simulink model "Simulering"  (R2021a)
settings: Solver=FixedStepDiscrete  StartTime=0.0  StopTime=100  FixedStep=0.0001  RelTol=1e-3
values from neighbouring files (symbols this model uses):
  D = 0.18    [grasklippare.m]
  L = 0.225    [grasklippare.m]
  r = 0.049    [grasklippare.m]
undefined symbols (not defined in the file or in its folder): DiscIntNeverNeededParam
libraries: simulink x4, pid_lib x3
settings Model: Creator=trane  LastModifiedBy=trane
settings SolverCC: AutoInsertRateTranBlk=on

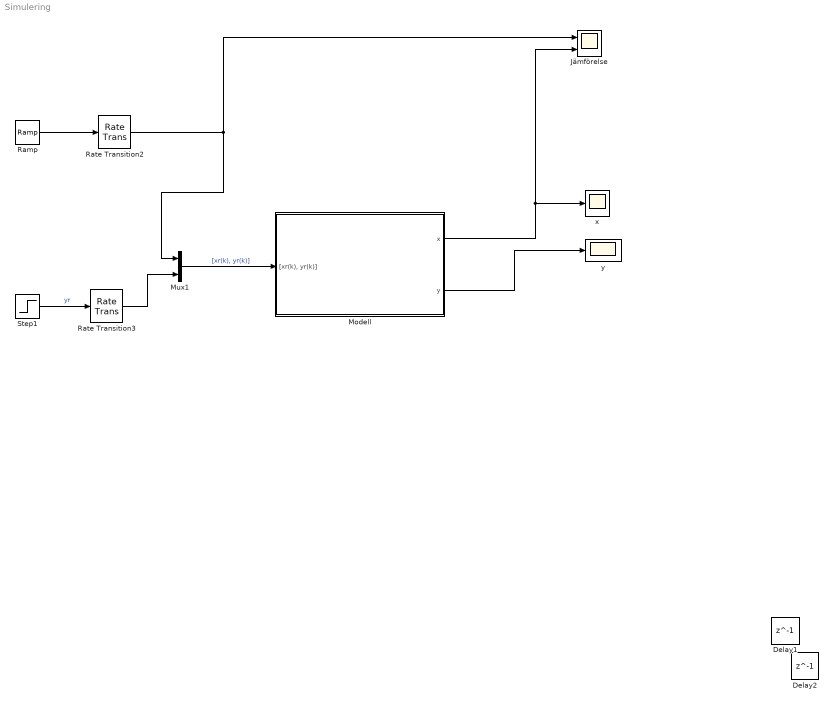
== system Simulering ==
  Delay1 : Delay  DelayLength=1  InitialCondition=0
  Delay2 : Delay  DelayLength=1  InitialCondition=0
  Jämförelse : Scope  NumInputPorts=2
  Modell : Subsystem
      mask Display: image('C:\Users\trane\OneDrive\Dokument\Kandidatarbete\Modell 550.jpg'); % Use "Edit Image" on toolstrip to change.
  Mux1 : Mux  Inputs=2
  Ramp : simulink/Sources/Ramp  slope=1  start=0  InitialOutput=0
  Rate Transition2 : RateTransition  OutPortSampleTime=0.02
  Rate Transition3 : RateTransition  OutPortSampleTime=0.02
  Step1 : Step  After=0  SampleTime=0.1
  x : Scope
  y : Scope
  wires:
  Mux1/1 -> Modell/1("[xr(k), yr(k)]")  "[xr(k), yr(k)]"
  Step1/1 -> Rate Transition3/1  "yr"
  Rate Transition2/1 -> Jämförelse/1, Mux1/1
  Rate Transition3/1 -> Mux1/2
  Ramp/1 -> Rate Transition2/1
  Modell/1(x) -> x/1, Jämförelse/2
  Modell/2(y) -> y/1

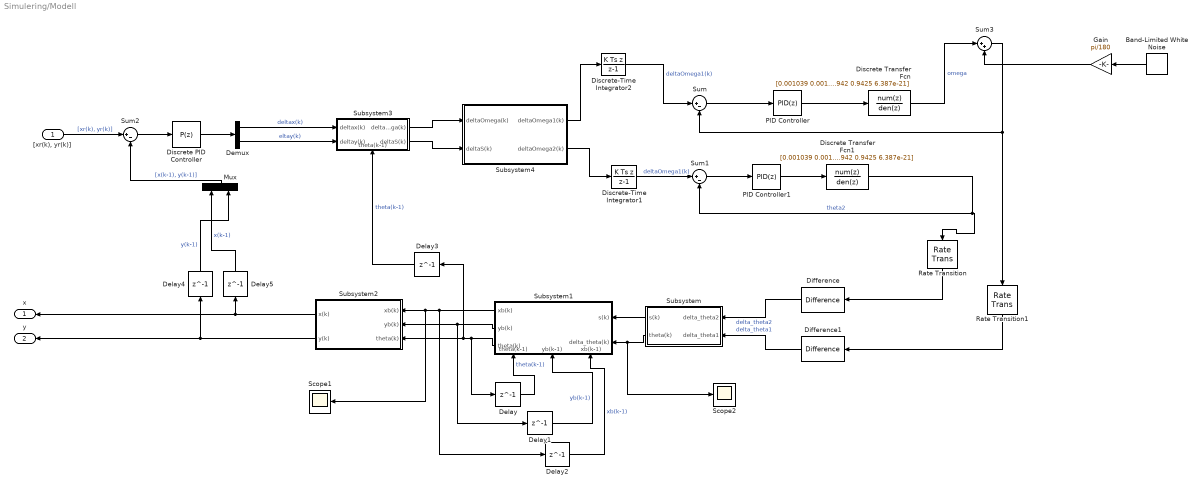
== system Simulering/Modell ==
  "[xr(k), yr(k)]" : Inport
  Band-Limited White Noise : simulink/Sources/Band-Limited White Noise  Cov=[0.001]  Ts=0.001  seed=[23341]
  Delay{,1..5} (6 alike) : Delay  DelayLength=1  InitialCondition=0
  Demux : Demux  Outputs=2
  Difference : simulink/Discrete/Difference  ICPrevInput=0.0  OutMin=[]  OutMax=[]  OutDataType=fixdt(1, 16)  OutScaling=2^-10  DoSatur=off
  Difference1 : simulink/Discrete/Difference  ICPrevInput=0.0  OutMin=[]  OutMax=[]  OutDataType=fixdt(1, 16)  OutScaling=2^-10  DoSatur=off
  Discrete Transfer Fcn : DiscreteTransferFcn  Numerator=[0.001039 0.001021 9.454e-10]  Denominator=[1 -1.942 0.9425 6.387e-21]  SampleTime=0.001
  Discrete Transfer Fcn1 : DiscreteTransferFcn  Numerator=[0.001039 0.001021 9.454e-10]  Denominator=[1 -1.942 0.9425 6.387e-21]  SampleTime=0.001
  Discrete PID Controller : pid_lib/PID Controller  Controller=P  Form=Parallel  TimeDomain=Discrete-time  UseExternalTs=off  SampleTime=-1  IntegratorMethod=Forward Euler  FilterMethod=Forward Euler  ControllerParametersSource=internal  P=10  I=1  D=0  UseFilter=on  N=100  TunerSelectOption=Transfer Function Based (PID Tuner App)  InitialConditionSource=internal  InitialConditionForIntegrator=0  InitialConditionForFilter=0  DifferentiatorICPrevScaledInput=0  ExternalReset=none  TrackingMode=off  Kt=1  LimitOutput=off  SatLimitsSource=internal  UpperSaturationLimit=inf  LowerSaturationLimit=-inf  LinearizeAsGain=off  AntiWindupMode=none  Kb=1  POutMin=[]  POutMax=[]  IOutMin=[]  IOutMax=[]  DOutMin=[]  DOutMax=[]  NOutMin=[]  NOutMax=[]  SumOutMin=[]  SumOutMax=[]  SaturationOutMin=[]  SaturationOutMax=[]  PParamMin=[]  PParamMax=[]  IParamMin=[]  IParamMax=[]  DParamMin=[]  DParamMax=[]  NParamMin=[]  NParamMax=[]  KbParamMin=[]  KbParamMax=[]  KtParamMin=[]  KtParamMax=[]  KbOutMin=[]  KbOutMax=[]  KtOutMin=[]  KtOutMax=[]  IntegratorOutMin=[]  IntegratorOutMax=[]  FilterOutMin=[]  FilterOutMax=[]  SumI1OutMin=[]  SumI1OutMax=[]  SumI2OutMin=[]  SumI2OutMax=[]  SumI3OutMin=[]  SumI3OutMax=[]  SumI4OutMin=[]  SumI4OutMax=[]  SumDOutMin=[]  SumDOutMax=[]  DifferentiatorOutMin=[]  DifferentiatorOutMax=[]  FilterDiffOutCoefMin=[]  FilterDiffOutCoefMax=[]  ReciprocalOutMin=[]  ReciprocalOutMax=[]  SumDenOutMin=[]  SumDenOutMax=[]  SumNumOutMin=[]  SumNumOutMax=[]  DivideOutMin=[]  DivideOutMax=[]  UdiffTsProdOutMin=[]  UdiffTsProdOutMax=[]  NTsProdOutMin=[]  NTsProdOutMax=[]  UintegralTsProdOutMin=[]  UintegralTsProdOutMax=[]  UngainTsProdOutMin=[]  UngainTsProdOutMax=[]  IntegratorContinuousStateAttributes=''  IntegratorStateMustResolveToSignalObject=off  IntegratorRTWStateStorageClass=Auto  FilterContinuousStateAttributes=''  FilterStateMustResolveToSignalObject=off  FilterRTWStateStorageClass=Auto  ParallelPVariant=InternalParameters  IdealPVariant=Disabled  IVariant=Disabled  DVariant=Disabled  IntegratorVariant=Disabled  SatVariant=Disabled  AWVariant=Disabled  PCopyVariant=Disabled  TRVariant=Disabled  FdbkBlocksVariant=Forward  IdealPFdbkVariant=Disabled  SatFdbkVariant=Disabled  DerivativeFilterVariant=Disabled  NVariant=Disabled  NCopyVariant=Disabled_SignalSpec  FilterICVariant=Disabled  IntegratorICVariant=Disabled  ExternalResetVariant=Disabled  TRSumVariant=Passthrough  SumFdbkVariant=Disabled  SumVariant=Passthrough_P  TsampFilterVariant=InternalTs  TsampNgainVariant=Passthrough  TsampIntegralVariant=Disabled_SignalSpec  ExternalSaturationOutDataTypeStr=Inherit: Same as second input
  Discrete-Time Integrator1 : DiscreteIntegrator  IntegratorMethod=Integration: Backward Euler  SampleTime=0.02  ICPrevOutput=DiscIntNeverNeededParam  ICPrevScaledInput=DiscIntNeverNeededParam
  Discrete-Time Integrator2 : DiscreteIntegrator  IntegratorMethod=Integration: Backward Euler  SampleTime=0.02  ICPrevOutput=DiscIntNeverNeededParam  ICPrevScaledInput=DiscIntNeverNeededParam
  Gain : Gain  Gain=pi/180
  Mux : Mux  Inputs=2
  PID Controller : pid_lib/PID Controller  Controller=PID  Form=Parallel  TimeDomain=Discrete-time  UseExternalTs=off  SampleTime=0.001  IntegratorMethod=Forward Euler  FilterMethod=Forward Euler  ControllerParametersSource=internal  P=10  I=20  D=0.3  UseFilter=on  N=50  TunerSelectOption=Transfer Function Based (PID Tuner App)  InitialConditionSource=internal  InitialConditionForIntegrator=0  InitialConditionForFilter=0  DifferentiatorICPrevScaledInput=0  ExternalReset=none  TrackingMode=off  Kt=1  LimitOutput=off  SatLimitsSource=internal  UpperSaturationLimit=inf  LowerSaturationLimit=-inf  LinearizeAsGain=on  AntiWindupMode=none  Kb=1  POutMin=[]  POutMax=[]  IOutMin=[]  IOutMax=[]  DOutMin=[]  DOutMax=[]  NOutMin=[]  NOutMax=[]  SumOutMin=[]  SumOutMax=[]  SaturationOutMin=[]  SaturationOutMax=[]  PParamMin=[]  PParamMax=[]  IParamMin=[]  IParamMax=[]  DParamMin=[]  DParamMax=[]  NParamMin=[]  NParamMax=[]  KbParamMin=[]  KbParamMax=[]  KtParamMin=[]  KtParamMax=[]  KbOutMin=[]  KbOutMax=[]  KtOutMin=[]  KtOutMax=[]  IntegratorOutMin=[]  IntegratorOutMax=[]  FilterOutMin=[]  FilterOutMax=[]  SumI1OutMin=[]  SumI1OutMax=[]  SumI2OutMin=[]  SumI2OutMax=[]  SumI3OutMin=[]  SumI3OutMax=[]  SumI4OutMin=[]  SumI4OutMax=[]  SumDOutMin=[]  SumDOutMax=[]  DifferentiatorOutMin=[]  DifferentiatorOutMax=[]  FilterDiffOutCoefMin=[]  FilterDiffOutCoefMax=[]  ReciprocalOutMin=[]  ReciprocalOutMax=[]  SumDenOutMin=[]  SumDenOutMax=[]  SumNumOutMin=[]  SumNumOutMax=[]  DivideOutMin=[]  DivideOutMax=[]  UdiffTsProdOutMin=[]  UdiffTsProdOutMax=[]  NTsProdOutMin=[]  NTsProdOutMax=[]  UintegralTsProdOutMin=[]  UintegralTsProdOutMax=[]  UngainTsProdOutMin=[]  UngainTsProdOutMax=[]  IntegratorContinuousStateAttributes=''  IntegratorStateMustResolveToSignalObject=off  IntegratorRTWStateStorageClass=Auto  FilterContinuousStateAttributes=''  FilterStateMustResolveToSignalObject=off  FilterRTWStateStorageClass=Auto  ParallelPVariant=InternalParameters  IdealPVariant=Disabled  IVariant=InternalParameters  DVariant=InternalParameters  IntegratorVariant=Discrete  SatVariant=Disabled  AWVariant=Passthrough  PCopyVariant=Disabled  TRVariant=Disabled  FdbkBlocksVariant=Forward  IdealPFdbkVariant=Disabled  SatFdbkVariant=Disabled  DerivativeFilterVariant=ForwardEulerFilter  NVariant=InternalParameters  NCopyVariant=Disabled  FilterICVariant=InternalICsFilter  IntegratorICVariant=InternalICs  ExternalResetVariant=Disabled  TRSumVariant=Passthrough  SumFdbkVariant=Disabled  SumVariant=Sum_PID  TsampFilterVariant=InternalTs  TsampNgainVariant=Passthrough  TsampIntegralVariant=Passthrough  ExternalSaturationOutDataTypeStr=Inherit: Same as second input
  PID Controller1 : pid_lib/PID Controller  Controller=PID  Form=Parallel  TimeDomain=Discrete-time  UseExternalTs=off  SampleTime=0.001  IntegratorMethod=Forward Euler  FilterMethod=Forward Euler  ControllerParametersSource=internal  P=10  I=20  D=0.3  UseFilter=on  N=50  TunerSelectOption=Transfer Function Based (PID Tuner App)  InitialConditionSource=internal  InitialConditionForIntegrator=0  InitialConditionForFilter=0  DifferentiatorICPrevScaledInput=0  ExternalReset=none  TrackingMode=off  Kt=1  LimitOutput=off  SatLimitsSource=internal  UpperSaturationLimit=inf  LowerSaturationLimit=-inf  LinearizeAsGain=on  AntiWindupMode=none  Kb=1  POutMin=[]  POutMax=[]  IOutMin=[]  IOutMax=[]  DOutMin=[]  DOutMax=[]  NOutMin=[]  NOutMax=[]  SumOutMin=[]  SumOutMax=[]  SaturationOutMin=[]  SaturationOutMax=[]  PParamMin=[]  PParamMax=[]  IParamMin=[]  IParamMax=[]  DParamMin=[]  DParamMax=[]  NParamMin=[]  NParamMax=[]  KbParamMin=[]  KbParamMax=[]  KtParamMin=[]  KtParamMax=[]  KbOutMin=[]  KbOutMax=[]  KtOutMin=[]  KtOutMax=[]  IntegratorOutMin=[]  IntegratorOutMax=[]  FilterOutMin=[]  FilterOutMax=[]  SumI1OutMin=[]  SumI1OutMax=[]  SumI2OutMin=[]  SumI2OutMax=[]  SumI3OutMin=[]  SumI3OutMax=[]  SumI4OutMin=[]  SumI4OutMax=[]  SumDOutMin=[]  SumDOutMax=[]  DifferentiatorOutMin=[]  DifferentiatorOutMax=[]  FilterDiffOutCoefMin=[]  FilterDiffOutCoefMax=[]  ReciprocalOutMin=[]  ReciprocalOutMax=[]  SumDenOutMin=[]  SumDenOutMax=[]  SumNumOutMin=[]  SumNumOutMax=[]  DivideOutMin=[]  DivideOutMax=[]  UdiffTsProdOutMin=[]  UdiffTsProdOutMax=[]  NTsProdOutMin=[]  NTsProdOutMax=[]  UintegralTsProdOutMin=[]  UintegralTsProdOutMax=[]  UngainTsProdOutMin=[]  UngainTsProdOutMax=[]  IntegratorContinuousStateAttributes=''  IntegratorStateMustResolveToSignalObject=off  IntegratorRTWStateStorageClass=Auto  FilterContinuousStateAttributes=''  FilterStateMustResolveToSignalObject=off  FilterRTWStateStorageClass=Auto  ParallelPVariant=InternalParameters  IdealPVariant=Disabled  IVariant=InternalParameters  DVariant=InternalParameters  IntegratorVariant=Discrete  SatVariant=Disabled  AWVariant=Passthrough  PCopyVariant=Disabled  TRVariant=Disabled  FdbkBlocksVariant=Forward  IdealPFdbkVariant=Disabled  SatFdbkVariant=Disabled  DerivativeFilterVariant=ForwardEulerFilter  NVariant=InternalParameters  NCopyVariant=Disabled  FilterICVariant=InternalICsFilter  IntegratorICVariant=InternalICs  ExternalResetVariant=Disabled  TRSumVariant=Passthrough  SumFdbkVariant=Disabled  SumVariant=Sum_PID  TsampFilterVariant=InternalTs  TsampNgainVariant=Passthrough  TsampIntegralVariant=Passthrough  ExternalSaturationOutDataTypeStr=Inherit: Same as second input
  Rate Transition : RateTransition  OutPortSampleTime=0.02
  Rate Transition1 : RateTransition  OutPortSampleTime=0.02
  Scope1 : Scope
  Scope2 : Scope
  Subsystem : Subsystem
  Subsystem1 : Subsystem
      settings: PortSchema="{\"entries\":[{\"content\":{\"sides\":[{\"content\":{\"connectorIds\":[\"In1\",\"In2\"]},\"type\":\"ConnectorPlacement.EquallySpacedRectSide\",\"uuid\":\"e0bb592b-54b6-434c-ba9d-c91d39128bfa\"},{\"content\":{\"connectorIds\":[\"Out1\",\"Out2\",\"Out3\"],\"side\":\"RIGHT\"},\"type\":\"ConnectorPlacement.EquallySpacedRectSide\",\"uuid\":\"5e9b4e58-2be4-4073-ab91-5d6ee9742bf3\"},{\"content\":{\"connectorIds\":[],\"side\":\"TOP\"},\"type\":\"ConnectorPlacement.EquallySpacedRectSide\",\"uuid\":\"d3f4358d-1cfc-4d0e-affe-c01d1bcf5e81\"},{\"content\":{\"connectorIds\":[\"In3\",\"In4\",\"In5\"],\"side\":\"BOTTOM\"},\"type\":\"ConnectorPlacement.EquallySpacedRectSide\",\"uuid\":\"cdd939dd-44d3-43db-8420-35e4dc5e28f9\"}]},\"type\":\"ConnectorPlacement.EquallySpacedConnector\",\"uuid\":\"c08356bc-bfa8-49e2-b64c-215d74b80249\"}],\"packageUris\":[\"http://schema.mathworks.com/mf0/Connector/R2020b\"],\"version\":\"1.0\"}"
  Subsystem2 : Subsystem
  Subsystem3 : Subsystem
      settings: PortSchema="{\"entries\":[{\"content\":{\"sides\":[{\"content\":{\"connectorIds\":[\"In1\",\"In2\"]},\"type\":\"ConnectorPlacement.EquallySpacedRectSide\",\"uuid\":\"b4f952da-16c3-4c71-9ec3-97babbcee399\"},{\"content\":{\"connectorIds\":[\"Out1\",\"Out2\"],\"side\":\"RIGHT\"},\"type\":\"ConnectorPlacement.EquallySpacedRectSide\",\"uuid\":\"a38d3374-2fce-4cc9-a5d0-4a9c8da8895b\"},{\"content\":{\"connectorIds\":[],\"side\":\"TOP\"},\"type\":\"ConnectorPlacement.EquallySpacedRectSide\",\"uuid\":\"ea42617f-bc21-41b8-85dc-e7b9436f5014\"},{\"content\":{\"connectorIds\":[\"In3\"],\"side\":\"BOTTOM\"},\"type\":\"ConnectorPlacement.EquallySpacedRectSide\",\"uuid\":\"b503501d-ebe3-468c-ae9d-fdcfa03b9079\"}]},\"type\":\"ConnectorPlacement.EquallySpacedConnector\",\"uuid\":\"87fb8522-e15d-4dff-ae71-18680433187a\"}],\"packageUris\":[\"http://schema.mathworks.com/mf0/Connector/R2020b\"],\"version\":\"1.0\"}"
  Subsystem4 : Subsystem
  Sum : Sum  Inputs=|+-
  Sum1 : Sum  Inputs=|+-
  Sum2 : Sum  Inputs=|+-
  Sum3 : Sum  Inputs=|++
  x : Outport
  y : Outport  Port=2
  wires:
  Delay1/1 -> Subsystem1/4(yb(k-1))  "yb(k-1)"
  Discrete-Time Integrator2/1 -> Sum/1  "deltaOmega1(k)"
  Subsystem1/1(xb(k)) -> Delay2/1, Scope1/1, Subsystem2/1(xb(k))
  Rate Transition1/1 -> Difference1/1
  Subsystem/2(theta(k)) -> Scope2/1, Subsystem1/2(delta_theta(k))
  Subsystem4/1(deltaOmega1(k)) -> Discrete-Time Integrator2/1
  PID Controller/1 -> Discrete Transfer Fcn/1
  Delay5/1 -> Mux/1  "x(k-1)"
  Demux/2 -> Subsystem3/2(deltay(k))  "eltay(k)"
  Subsystem3/2(deltaS(k)) -> Subsystem4/2(deltaS(k))
  Demux/1 -> Subsystem3/1(deltax(k))  "deltax(k)"
  Discrete-Time Integrator1/1 -> Sum1/1  "deltaOmega1(k)"
  Subsystem2/2(y(k)) -> y/1, Delay4/1
  Difference/1 -> Subsystem/1(delta_theta2)  "delta_theta2"
  Discrete Transfer Fcn1/1 -> Rate Transition/1, Sum1/2  "theta2"
  Delay3/1 -> Subsystem3/3(theta(k-1))  "theta(k-1)"
  Subsystem4/2(deltaOmega2(k)) -> Discrete-Time Integrator1/1
  Subsystem3/1(deltaOmega(k)) -> Subsystem4/1(deltaOmega(k))
  Subsystem1/2(yb(k)) -> Delay1/1, Subsystem2/2(yb(k))
  "[xr(k), yr(k)]"/1 -> Sum2/1  "[xr(k), yr(k)]"
  Subsystem1/3(theta(k)) -> Delay3/1, Subsystem2/3(theta(k)), Delay/1
  PID Controller1/1 -> Discrete Transfer Fcn1/1
  Sum1/1 -> PID Controller1/1
  Delay4/1 -> Mux/2  "y(k-1)"
  Sum/1 -> PID Controller/1
  Rate Transition/1 -> Difference/1
  Delay/1 -> Subsystem1/5(theta(k-1))  "theta(k-1)"
  Delay2/1 -> Subsystem1/3(xb(k-1))  "xb(k-1)"
  Subsystem/1(s(k)) -> Subsystem1/1(s(k))
  Mux/1 -> Sum2/2  "[x(k-1), y(k-1)]"
  Subsystem2/1(x(k)) -> x/1, Delay5/1
  Difference1/1 -> Subsystem/2(delta_theta1)  "delta_theta1"
  Discrete Transfer Fcn/1 -> Sum3/1  "omega"
  Sum3/1 -> Sum/2, Rate Transition1/1
  Gain/1 -> Sum3/2
  Band-Limited White Noise/1 -> Gain/1
  Sum2/1 -> Discrete PID Controller/1
  Discrete PID Controller/1 -> Demux/1

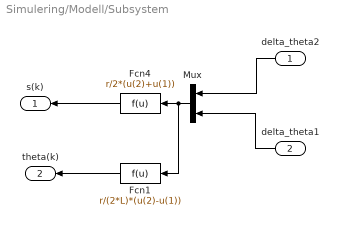
== system Simulering/Modell/Subsystem ==
  delta_theta2 : Inport
  delta_theta1 : Inport  Port=2
  Fcn1 : Fcn  Expr=r/(2*L)*(u(2)-u(1))
  Fcn4 : Fcn  Expr=r/2*(u(2)+u(1))
  Mux : Mux  Inputs=2
  s(k) : Outport
  theta(k) : Outport  Port=2
  wires:
  delta_theta2/1 -> Mux/1
  delta_theta1/1 -> Mux/2
  Mux/1 -> Fcn1/1, Fcn4/1
  Fcn4/1 -> s(k)/1
  Fcn1/1 -> theta(k)/1

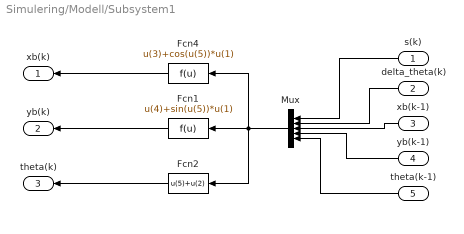
== system Simulering/Modell/Subsystem1 ==
  s(k) : Inport
  delta_theta(k) : Inport  Port=2
  xb(k-1) : Inport  Port=3
  yb(k-1) : Inport  Port=4
  theta(k-1) : Inport  Port=5
  Fcn1 : Fcn  Expr=u(4)+sin(u(5))*u(1)
  Fcn2 : Fcn  Expr=u(5)+u(2)
  Fcn4 : Fcn  Expr=u(3)+cos(u(5))*u(1)
  Mux : Mux  Inputs=5
  xb(k) : Outport
  yb(k) : Outport  Port=2
  theta(k) : Outport  Port=3
  wires:
  Mux/1 -> Fcn2/1, Fcn1/1, Fcn4/1
  s(k)/1 -> Mux/1
  delta_theta(k)/1 -> Mux/2
  xb(k-1)/1 -> Mux/3
  yb(k-1)/1 -> Mux/4
  theta(k-1)/1 -> Mux/5
  Fcn4/1 -> xb(k)/1
  Fcn1/1 -> yb(k)/1
  Fcn2/1 -> theta(k)/1

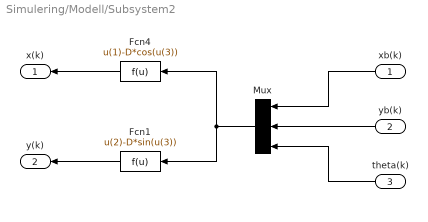
== system Simulering/Modell/Subsystem2 ==
  xb(k) : Inport
  yb(k) : Inport  Port=2
  theta(k) : Inport  Port=3
  Fcn1 : Fcn  Expr=u(2)-D*sin(u(3))
  Fcn4 : Fcn  Expr=u(1)-D*cos(u(3))
  Mux : Mux  Inputs=3
  x(k) : Outport
  y(k) : Outport  Port=2
  wires:
  xb(k)/1 -> Mux/1
  yb(k)/1 -> Mux/2
  theta(k)/1 -> Mux/3
  Fcn4/1 -> x(k)/1
  Mux/1 -> Fcn1/1, Fcn4/1
  Fcn1/1 -> y(k)/1

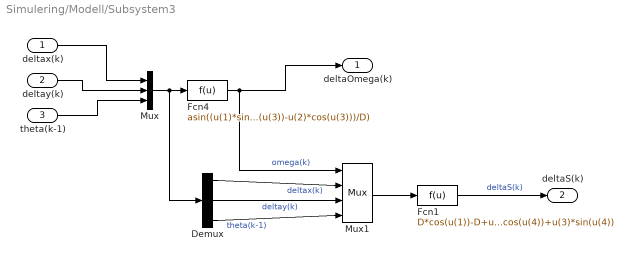
== system Simulering/Modell/Subsystem3 ==
  deltax(k) : Inport
  deltay(k) : Inport  Port=2
  theta(k-1) : Inport  Port=3
  Demux : Demux  Outputs=3
  Fcn1 : Fcn  Expr=D*cos(u(1))-D+u(2)*cos(u(4))+u(3)*sin(u(4))
  Fcn4 : Fcn  Expr=asin((u(1)*sin(u(3))-u(2)*cos(u(3)))/D)
  Mux : Mux  Inputs=3
  Mux1 : Mux
  deltaOmega(k) : Outport
  deltaS(k) : Outport  Port=2
  wires:
  deltax(k)/1 -> Mux/1
  deltay(k)/1 -> Mux/2
  theta(k-1)/1 -> Mux/3
  Mux/1 -> Demux/1, Fcn4/1
  Fcn4/1 -> Mux1/1, deltaOmega(k)/1  "omega(k)"
  Demux/1 -> Mux1/2  "deltax(k)"
  Demux/3 -> Mux1/4  "theta(k-1)"
  Demux/2 -> Mux1/3  "deltay(k)"
  Mux1/1 -> Fcn1/1
  Fcn1/1 -> deltaS(k)/1  "deltaS(k)"

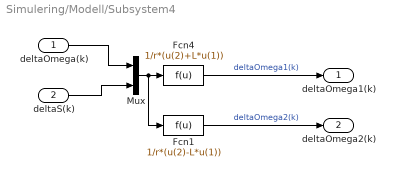
== system Simulering/Modell/Subsystem4 ==
  deltaOmega(k) : Inport
  deltaS(k) : Inport  Port=2
  Fcn1 : Fcn  Expr=1/r*(u(2)-L*u(1))
  Fcn4 : Fcn  Expr=1/r*(u(2)+L*u(1))
  Mux : Mux  Inputs=2
  deltaOmega1(k) : Outport
  deltaOmega2(k) : Outport  Port=2
  wires:
  deltaOmega(k)/1 -> Mux/1
  deltaS(k)/1 -> Mux/2
  Mux/1 -> Fcn1/1, Fcn4/1
  Fcn4/1 -> deltaOmega1(k)/1  "deltaOmega1(k)"
  Fcn1/1 -> deltaOmega2(k)/1  "deltaOmega2(k)"
